simulink model "grzanie"  (R2015a)
settings: Solver=ode4  StartTime=0.0  StopTime=600  FixedStep=0.1  RelTol=1e-3
undefined symbols (not defined in the file): sigbuilder_block
settings Model: Creator=Student  LastModifiedBy=lenovo

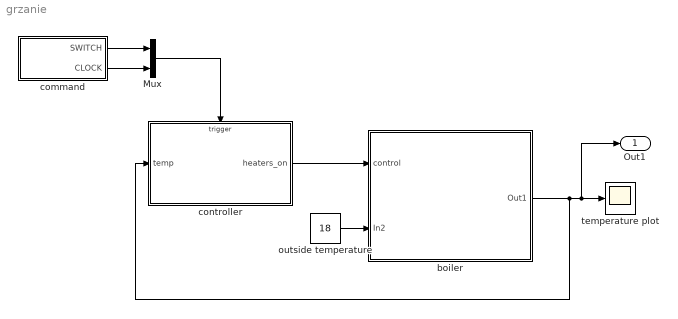
== system grzanie ==
  Mux : Mux  Inputs=2
  "boiler " : Subsystem
  command : Subsystem  Tag=STV Subsys  LoadFcn=sigbuilder_block('load');  StartFcn=sigbuilder_block('start');  StopFcn=sigbuilder_block('stop');  ClipboardFcn=sigbuilder_block('clipboard');  mask(Sigbuilder block){}
      mask help: Simulink:masks:SigbuilderBlock_MD
      mask init:
      | if ~strcmp(get_param(bdroot(gcbh),'SimulationStatus'),'stopped') tuvar = sigbuilder_block('maskInit'); end
      settings: CopyFcn=sigbuilder_block('copy');  DeleteFcn=sigbuilder_block('delete');  ModelCloseFcn=sigbuilder_block('modelClose');  PreSaveFcn=sigbuilder_block('preSave');  PauseFcn=sigbuilder_block('pause');  ContinueFcn=sigbuilder_block('continue');  NameChangeFcn=sigbuilder_block('namechange');  OpenFcn=sigbuilder_block('open',[437.6 199.2 550.4 400 ]);  CloseFcn=sigbuilder_block('close');
      mask Display: plot(0, 0, 100, 100,[2, 2, 32, 32, 2], [68, 8, 8, 68, 68],[32, 2], [38, 38], [32, 19, 2],[53, 60, 44], [32, 17, 17, 2],[16, 16, 31, 31]);txt = getActiveGroup(gcbh);text(2, 100, txt,'verticalAlignment', 'top');
  controller : Stateflow chart  TreatAsAtomicUnit=on
  outside temperature : Constant  Value=18
  temperature plot : Scope
      settings: TimeRange=499.9  YMin=10  YMax=18
  Out1 : Outport
  wires:
  outside temperature/1 -> "boiler "/2(In2)
  "boiler "/1(Out1) -> controller/1(temp), Out1/1, temperature plot/1
  Mux/1 -> controller/Trigger
  command/1(SWITCH) -> Mux/1
  controller/1(heaters_on) -> "boiler "/1(control)
  command/2(CLOCK) -> Mux/2

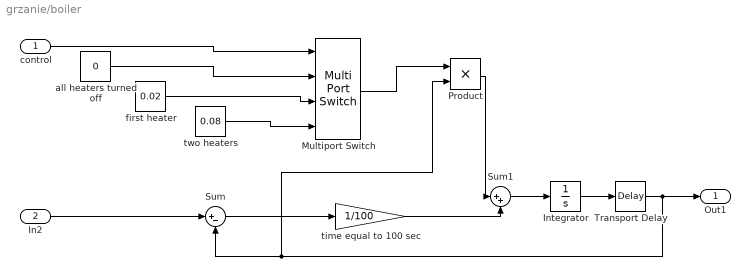
== system grzanie/boiler  ==
  control : Inport
  In2 : Inport  Port=2
  Integrator : Integrator
  Multiport Switch : MultiPortSwitch  DataPortOrder=Zero-based contiguous
  Product : Product
  Sum : Sum  Inputs=|+-
  Sum1 : Sum  Inputs=|++
  Transport Delay : TransportDelay
  "all heaters turned off " : Constant  Value=0
  first heater : Constant  Value=0.02
  time equal to 100 sec : Gain  Gain=1/100
  two heaters : Constant  Value=0.08
  Out1 : Outport
  wires:
  Sum/1 -> time equal to 100 sec/1
  In2/1 -> Sum/1
  Product/1 -> Sum1/1
  Sum1/1 -> Integrator/1
  time equal to 100 sec/1 -> Sum1/2
  Integrator/1 -> Transport Delay/1
  Transport Delay/1 -> Out1/1, Product/2, Sum/2
  control/1 -> Multiport Switch/1
  "all heaters turned off "/1 -> Multiport Switch/2
  first heater/1 -> Multiport Switch/3
  two heaters/1 -> Multiport Switch/4
  Multiport Switch/1 -> Product/1

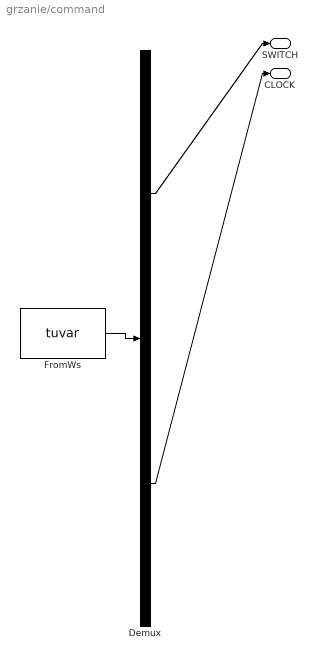
== system grzanie/command ==
  Demux : Demux  Tag=STV Demux  Outputs=2
  FromWs : FromWorkspace  Tag=STV FromWs  VariableName=tuvar  SampleTime=0
      SigBuilderData=|
      | common.afterFinalStr = 'Extrapolate'
      | common.sampleTime = 0
      | dataSet.timeRange = [0 600]
      | dataSet.name = 'Group 1'
      | sbobj.Groups.Name = 'Group 1'
      | sbobj.Groups.Signals(1).Name = 'SWITCH'
      | sbobj.Groups.Signals(1).XData = [0 150 150 300 300 450 450 600]
      | sbobj.Groups.Signals(1).YData = [0 0 1 1 0 0 1 1]
      | sbobj.Groups.Signals(2).Name = 'CLOCK'
      | sbobj.Groups.Signals(2).XData = [0 0.5 0.5 1 1 1.5 1.5 2 2 2.5 2.5 3 ... (2397 elements, 1x2397)]
      | sbobj.Groups.Signals(2).YData = [2 2 -2 -2 2 2 -2 -2 2 2 -2 -2 ... (2397 elements, 1x2397)]
      | sbobj.Groups.TimeRange = [0 600]
  SWITCH : Outport  Tag=STV Outport
  CLOCK : Outport  Tag=STV Outport  Port=2
  wires:
  FromWs/1 -> Demux/1
  Demux/1 -> SWITCH/1
  Demux/2 -> CLOCK/1

== stateflow chart grzanie/controller ==
  state PowerOn
    state Heater1 [parallel]
      settings: executionOrder=1
      state On
      state Off
      PowerOn.Heater1.On -> PowerOn.Heater1.Off : [temp>70]
      (default) -> PowerOn.Heater1.Off
      PowerOn.Heater1.Off -> PowerOn.Heater1.On : [temp<=70]
    state Heater2 [parallel]
      settings: executionOrder=2
      state On
      state Off
      PowerOn.Heater2.On -> PowerOn.Heater2.Off : [temp>40]
      (default) -> PowerOn.Heater2.Off
      PowerOn.Heater2.Off -> PowerOn.Heater2.On : [temp<=40]
    state HeatersOn [parallel]
      during: heaters_on=in(Heater1.On)+in(Heater2.On);
      settings: executionOrder=3
  state PowerOff
    entry: heaters_on=0;
  PowerOff -> PowerOn : SWITCH
  PowerOn -> PowerOff : SWITCH
  (default) -> PowerOff
  data: temp input; heaters_on output double
  events: SWITCH input EITHER_EDGE_EVENT; CLOCK input RISING_EDGE_EVENT
